simulink model "simschemeFun"  (R2019a)
settings: Solver=ode45  StartTime=0.0  StopTime=10  MaxStep=1e-4  RelTol=1e-3  EnableMultiTasking=on
values from neighbouring files (symbols this model uses):
  a = 0.2    [mainFun.m]    (also in mainFunTV.m)
  f2 = 5    [mainFun.m]    (also in mainFunTV.m)
  h = 1    [mainFun.m]    (also in mainFunTV.m; mainPID.m = 0.5)
  k = 5    [mainFun.m]    (also in mainFunTV.m)
  omega = 50    [mainFun.m]    (also in mainFunTV.m; mainPID.m = pi*[.8 .8 .8])
  theta0 = 0    [mainFun.m]    (also in mainFunTV.m)
settings Model: Creator=Adriano  LastModifiedBy=adria
settings DataIOCC: LimitDataPoints=on  SaveFormat=Array  ReturnWorkspaceOutputs=off
settings OptimizationCC: LifeSpan=inf
settings DebuggingCC: SFUnexpectedBacktrackingDiag=warning  SFNoUnconditionalDefaultTransitionDiag=warning  SFExecutionAtInitializationDiag=none  ArithmeticOperatorsInVariantConditions=warning
settings HardwareCC: ProdBitPerPointer=32  ProdBitPerSizeT=32  ProdBitPerPtrDiffT=32  ProdLargestAtomicFloat=None  ProdIntDivRoundTo=Undefined  ProdEndianess=Unspecified  ProdWordSize=32  ProdHWDeviceType=32-bit Generic
settings ModelReferenceCC: PropagateSignalLabelsOutOfModel=off
settings SFSimCC: SimUseLocalCustomCode=off
settings RTWCC: RTWUseLocalCustomCode=off
settings CodeAppCC: StateflowObjectComments=on
settings GRTTargetCC: TargetLangStandard=C89/C90 (ANSI)  GeneratePreprocessorConditionals=Disable all
settings ConfigComp: CovMetricSettings=dw  CovHtmlReporting=on  CovSaveCumulativeToWorkspaceVar=on  CovSaveSingleToWorkspaceVar=on  CovExternalEMLEnable=off

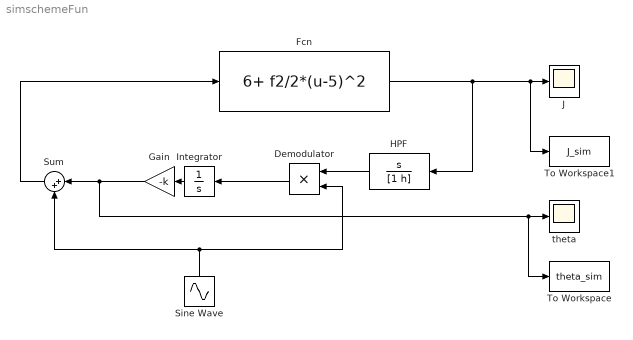
== system simschemeFun ==
  Demodulator : Product
  Fcn : Fcn  Expr=6+ f2/2*(u-5)^2
  Gain : Gain  Gain=-k
  HPF : TransferFcn  Numerator=[1 0]  Denominator=[1 h]
  Integrator : Integrator  InitialCondition=-theta0/k
  J : Scope
  Sine Wave : Sin  Amplitude=a  Frequency=omega  SampleTime=0
  Sum : Sum  Inputs=|++
  To Workspace : ToWorkspace  VariableName=theta_sim  SaveFormat=Structure With Time  SampleTime=-1
  To Workspace1 : ToWorkspace  VariableName=J_sim  SaveFormat=Structure With Time  SampleTime=-1
  theta : Scope
  wires:
  HPF/1 -> Demodulator/1
  Demodulator/1 -> Integrator/1
  Integrator/1 -> Gain/1
  Sine Wave/1 -> Demodulator/2, Sum/2
  Gain/1 -> To Workspace/1, theta/1, Sum/1
  Fcn/1 -> HPF/1, To Workspace1/1, J/1
  Sum/1 -> Fcn/1
